simulink model "PPSFB_DC_DC_att_11"  (R2021a)
settings: Solver=ode23t  StartTime=0.0  StopTime=0.5  FixedStep=1.0000e-8  RelTol=1e-3
libraries: spsSeriesRLCBranchLib x31, spsVoltageMeasurementLib x9, spsMosfetLib x8, spsGroundLib x6, spsControlledVoltageSourceLib x3, spsCurrentMeasurementLib x2, spsLinearTransformerLib x2, pid_lib x2, spsParallelRLCBranchLib x2, spsDCVoltageSourceLib x1, spspowerguiLib x1
settings Model: Creator=prizm  LastModifiedBy=prizm

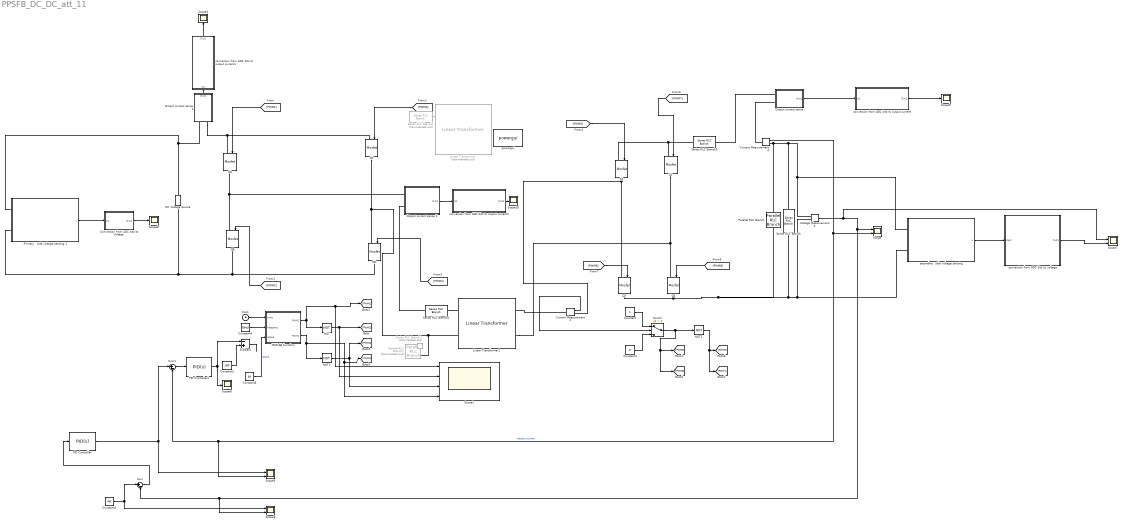
== system PPSFB_DC_DC_att_11 ==
  Clock : Clock
  Constant : Constant
  Constant1 : Constant  Value=0
  Constant2 : Constant  Value=180
  Constant3 : Constant  Value=48
  Constant4 : Constant  Value=65e3
  Constant5 : Constant  Value=90  SampleTime=1e-8
  "Conversion from ADC bits to Voltage " : Subsystem
  Current Measurement1 : spsCurrentMeasurementLib/Current Measurement  PhasorSimulation=off  OutputType=Complex  PSBequivalent=0
  Current Measurement4 : spsCurrentMeasurementLib/Current Measurement  PhasorSimulation=off  OutputType=Complex  PSBequivalent=0
  DC Voltage Source : spsDCVoltageSourceLib/DC Voltage Source  Amplitude=800  Measurements=None
  Linear Transformer : spsLinearTransformerLib/Linear Transformer  Commented=on  UNITS=SI  NominalPower=[5000 100000]  winding1=[750 0 0]  winding2=[107.25 0.003 300e-9]  ThreeWindings=off  winding3=[3.15e+05 0 0]  RmLm=[10e9 10.66e-3]  Measurements=None  DataType=on
  Linear Transformer1 : spsLinearTransformerLib/Linear Transformer  UNITS=SI  NominalPower=[5000 65000]  winding1=[800 0.245 10e-6]  winding2=[114 5e-3 1.143e-6]  ThreeWindings=off  winding3=[3.15e+05 0 0]  RmLm=[10e9 3.53e-3]  Measurements=None  DataType=on
  MATLAB Function : MATLAB Function  TreatAsAtomicUnit=on
  NOT : Logic  Operator=NOT  IconShape=distinctive  AllPortsSameDT=off  OutDataTypeStr=boolean
  NOT1 : Logic  Operator=NOT  IconShape=distinctive  AllPortsSameDT=off  OutDataTypeStr=boolean
  NOT2 : Logic  Operator=NOT  IconShape=distinctive  AllPortsSameDT=off  OutDataTypeStr=boolean
  "Output current sense " : Subsystem
  Output current sense 1 : Subsystem
  Output current sense 2 : Subsystem
  PID Controller : pid_lib/PID Controller  Controller=PID  Form=Parallel  TimeDomain=Continuous-time  UseExternalTs=off  SampleTime=-1  IntegratorMethod=Forward Euler  FilterMethod=Forward Euler  ControllerParametersSource=internal  P=0.003  I=100  D=0  UseFilter=on  N=100  TunerSelectOption=Frequency Response Based  InitialConditionSource=internal  InitialConditionForIntegrator=0  InitialConditionForFilter=0  DifferentiatorICPrevScaledInput=0  ExternalReset=none  TrackingMode=off  Kt=1  LimitOutput=on  SatLimitsSource=internal  UpperSaturationLimit=200  LowerSaturationLimit=0  LinearizeAsGain=on  AntiWindupMode=none  Kb=1  POutMin=[]  POutMax=[]  IOutMin=[]  IOutMax=[]  DOutMin=[]  DOutMax=[]  NOutMin=[]  NOutMax=[]  SumOutMin=[]  SumOutMax=[]  SaturationOutMin=[]  SaturationOutMax=[]  PParamMin=[]  PParamMax=[]  IParamMin=[]  IParamMax=[]  DParamMin=[]  DParamMax=[]  NParamMin=[]  NParamMax=[]  KbParamMin=[]  KbParamMax=[]  KtParamMin=[]  KtParamMax=[]  KbOutMin=[]  KbOutMax=[]  KtOutMin=[]  KtOutMax=[]  IntegratorOutMin=[]  IntegratorOutMax=[]  FilterOutMin=[]  FilterOutMax=[]  SumI1OutMin=[]  SumI1OutMax=[]  SumI2OutMin=[]  SumI2OutMax=[]  SumI3OutMin=[]  SumI3OutMax=[]  SumI4OutMin=[]  SumI4OutMax=[]  SumDOutMin=[]  SumDOutMax=[]  DifferentiatorOutMin=[]  DifferentiatorOutMax=[]  FilterDiffOutCoefMin=[]  FilterDiffOutCoefMax=[]  ReciprocalOutMin=[]  ReciprocalOutMax=[]  SumDenOutMin=[]  SumDenOutMax=[]  SumNumOutMin=[]  SumNumOutMax=[]  DivideOutMin=[]  DivideOutMax=[]  UdiffTsProdOutMin=[]  UdiffTsProdOutMax=[]  NTsProdOutMin=[]  NTsProdOutMax=[]  UintegralTsProdOutMin=[]  UintegralTsProdOutMax=[]  UngainTsProdOutMin=[]  UngainTsProdOutMax=[]  IntegratorContinuousStateAttributes=''  IntegratorStateMustResolveToSignalObject=off  IntegratorRTWStateStorageClass=Auto  FilterContinuousStateAttributes=''  FilterStateMustResolveToSignalObject=off  FilterRTWStateStorageClass=Auto  ParallelPVariant=InternalParameters  IdealPVariant=Disabled  IVariant=InternalParameters  DVariant=InternalParameters  IntegratorVariant=Continuous  SatVariant=Enabled  AWVariant=Passthrough  PCopyVariant=Disabled  TRVariant=Disabled  FdbkBlocksVariant=Forward  IdealPFdbkVariant=Disabled  SatFdbkVariant=Disabled  DerivativeFilterVariant=ContFilter  NVariant=InternalParameters  NCopyVariant=Disabled  FilterICVariant=InternalICsFilter  IntegratorICVariant=InternalICs  ExternalResetVariant=Disabled  TRSumVariant=Passthrough  SumFdbkVariant=Disabled  SumVariant=Sum_PID  TsampFilterVariant=InternalTs  TsampNgainVariant=Passthrough  TsampIntegralVariant=Passthrough  ExternalSaturationOutDataTypeStr=Inherit: Same as second input
  PID Controller1 : pid_lib/PID Controller  Controller=PID  Form=Parallel  TimeDomain=Continuous-time  UseExternalTs=off  SampleTime=-1  IntegratorMethod=Forward Euler  FilterMethod=Forward Euler  ControllerParametersSource=internal  P=0.074  I=942.478  D=0  UseFilter=on  N=100  TunerSelectOption=Transfer Function Based (PID Tuner App)  InitialConditionSource=internal  InitialConditionForIntegrator=0  InitialConditionForFilter=0  DifferentiatorICPrevScaledInput=0  ExternalReset=none  TrackingMode=off  Kt=1  LimitOutput=on  SatLimitsSource=internal  UpperSaturationLimit=180  LowerSaturationLimit=0  LinearizeAsGain=on  AntiWindupMode=none  Kb=1  POutMin=[]  POutMax=[]  IOutMin=[]  IOutMax=[]  DOutMin=[]  DOutMax=[]  NOutMin=[]  NOutMax=[]  SumOutMin=[]  SumOutMax=[]  SaturationOutMin=[]  SaturationOutMax=[]  PParamMin=[]  PParamMax=[]  IParamMin=[]  IParamMax=[]  DParamMin=[]  DParamMax=[]  NParamMin=[]  NParamMax=[]  KbParamMin=[]  KbParamMax=[]  KtParamMin=[]  KtParamMax=[]  KbOutMin=[]  KbOutMax=[]  KtOutMin=[]  KtOutMax=[]  IntegratorOutMin=[]  IntegratorOutMax=[]  FilterOutMin=[]  FilterOutMax=[]  SumI1OutMin=[]  SumI1OutMax=[]  SumI2OutMin=[]  SumI2OutMax=[]  SumI3OutMin=[]  SumI3OutMax=[]  SumI4OutMin=[]  SumI4OutMax=[]  SumDOutMin=[]  SumDOutMax=[]  DifferentiatorOutMin=[]  DifferentiatorOutMax=[]  FilterDiffOutCoefMin=[]  FilterDiffOutCoefMax=[]  ReciprocalOutMin=[]  ReciprocalOutMax=[]  SumDenOutMin=[]  SumDenOutMax=[]  SumNumOutMin=[]  SumNumOutMax=[]  DivideOutMin=[]  DivideOutMax=[]  UdiffTsProdOutMin=[]  UdiffTsProdOutMax=[]  NTsProdOutMin=[]  NTsProdOutMax=[]  UintegralTsProdOutMin=[]  UintegralTsProdOutMax=[]  UngainTsProdOutMin=[]  UngainTsProdOutMax=[]  IntegratorContinuousStateAttributes=''  IntegratorStateMustResolveToSignalObject=off  IntegratorRTWStateStorageClass=Auto  FilterContinuousStateAttributes=''  FilterStateMustResolveToSignalObject=off  FilterRTWStateStorageClass=Auto  ParallelPVariant=InternalParameters  IdealPVariant=Disabled  IVariant=InternalParameters  DVariant=InternalParameters  IntegratorVariant=Continuous  SatVariant=Enabled  AWVariant=Passthrough  PCopyVariant=Disabled  TRVariant=Disabled  FdbkBlocksVariant=Forward  IdealPFdbkVariant=Disabled  SatFdbkVariant=Disabled  DerivativeFilterVariant=ContFilter  NVariant=InternalParameters  NCopyVariant=Disabled  FilterICVariant=InternalICsFilter  IntegratorICVariant=InternalICs  ExternalResetVariant=Disabled  TRSumVariant=Passthrough  SumFdbkVariant=Disabled  SumVariant=Sum_PID  TsampFilterVariant=InternalTs  TsampNgainVariant=Passthrough  TsampIntegralVariant=Passthrough  ExternalSaturationOutDataTypeStr=Inherit: Same as second input
  Parallel RLC Branch : spsParallelRLCBranchLib/Parallel RLC Branch  LConnTagsString=a  RConnTagsString=__new0  BranchType=R  Resistance=0.461  Inductance=1e-3  SetiL0=off  InitialCurrent=0  Capacitance=1e-6  Setx0=off  InitialVoltage=0  Measurements=None
  Parallel RLC Branch1 : spsParallelRLCBranchLib/Parallel RLC Branch  Commented=on  LConnTagsString=a  RConnTagsString=__new0  BranchType=L  Resistance=100  Inductance=1.88e-6  SetiL0=off  InitialCurrent=0  Capacitance=1e-6  Setx0=off  InitialVoltage=0  Measurements=None
  Primary   side voltage sensing 1 : Subsystem
  Q{1..4} (4 alike) : spsMosfetLib/Mosfet  Ron=0.1  Lon=0  Rd=0.01  Vfd=2  IC=0  Rs=1e5  Cs=inf  Measurements=off
  QA : spsMosfetLib/Mosfet  Ron=0.1  Lon=0  Rd=0.01  Vfd=2  IC=0  Rs=1e5  Cs=inf  Measurements=off
  QB : spsMosfetLib/Mosfet  Ron=0.1  Lon=0  Rd=0.01  Vfd=2  IC=0  Rs=1e5  Cs=inf  Measurements=off
  QC : spsMosfetLib/Mosfet  Ron=0.1  Lon=0  Rd=0.01  Vfd=2  IC=0  Rs=1e5  Cs=inf  Measurements=off
  QD : spsMosfetLib/Mosfet  Ron=0.1  Lon=0  Rd=0.01  Vfd=2  IC=0  Rs=1e5  Cs=inf  Measurements=off
  Scope{,3,5,7} (4 alike) : Scope  NumInputPorts=2
  Scope1 : Scope  NumInputPorts=4
  Scope{4,6,8..10} (5 alike) : Scope
  Series RLC Branch : spsSeriesRLCBranchLib/Series RLC Branch  LConnTagsString=__new0  RConnTagsString=__new0  BranchType=C  Resistance=1  Inductance=1e-3  SetiL0=off  InitialCurrent=0  Capacitance=1e-3  Setx0=off  InitialVoltage=0  Measurements=None
  Series RLC Branch1 : spsSeriesRLCBranchLib/Series RLC Branch  Commented=on  LConnTagsString=__new0  RConnTagsString=__new0  BranchType=RL  Resistance=0.126  Inductance=10e-6  SetiL0=off  InitialCurrent=0  Capacitance=1e-6  Setx0=off  InitialVoltage=0  Measurements=None
  Series RLC Branch2 : spsSeriesRLCBranchLib/Series RLC Branch  Commented=on  LConnTagsString=__new0  RConnTagsString=__new0  BranchType=C  Resistance=1  Inductance=1e-3  SetiL0=off  InitialCurrent=0  Capacitance=200e-12  Setx0=off  InitialVoltage=0  Measurements=None
  Series RLC Branch3 : spsSeriesRLCBranchLib/Series RLC Branch  LConnTagsString=__new0  RConnTagsString=__new0  BranchType=L  Resistance=0.005  Inductance=10e-6  SetiL0=off  InitialCurrent=0  Capacitance=1e-6  Setx0=off  InitialVoltage=0  Measurements=None
  Series RLC Branch4 : spsSeriesRLCBranchLib/Series RLC Branch  LConnTagsString=__new0  RConnTagsString=__new0  BranchType=L  Resistance=1  Inductance=20e-6  SetiL0=off  InitialCurrent=0  Capacitance=1e-6  Setx0=off  InitialVoltage=0  Measurements=None
  Subtract : Sum  Inputs=-+
  Sum : Sum  Inputs=|+-
  Sum1 : Sum  Inputs=|+-
  Switch : Switch  Criteria=u2 > Threshold
  Voltage Measurement2 : spsVoltageMeasurementLib/Voltage Measurement  PhasorSimulation=off  OutputType=Complex  PSBequivalent=0
  conversion from ADC bits to output current : Subsystem
  conversion from ADC bits to output current1 : Subsystem
  conversion from ADC bits to output current2 : Subsystem
  "conversion from ADC bits to voltage " : Subsystem
  powergui : spspowerguiLib/powergui  Priority=1  SimulationMode=Discrete  SampleTime=1e-8  frequency=60  Iterations=50  frequencyindice=0  Pbase=100e6  ErrMax=1e-4  UnitsV=kV  UnitsW=MW  buscounter=0  FunctionMessages=off  echomessages=off  EnableUseOfTLC=off  CurrentSourceSwitches=off  DisableSnubberDevices=off  DisableRonSwitches=off  DisableVfSwitches=off  DisplayEquations=off  AutomaticDiscreteSolvers=off  SolverType=Tustin/Backward Euler (TBE)  Interpol=off  ExternalGateDelay=off  methode=off  Ts=100  x0status=blocks  SPID=on  SwTol=0  HookPort=off  NonlinearTolerance=1e-4  nMaxIteration=100  ContinueOnMaxIteration=off  RestoreLinks=warning  ResistiveCurrentMeasurement=off  Frange=[0:2:500]  Ylog=off  Xlog=on  ShowGrid=off  save=off  variable=ZData  structure=0  ZoomFFT=off  StartTime=0.0  cycles=1  DisplayStyle=1  fundamental=60  FreqAxis=off  MaxFrequency=1000  frequencyindicesteady=1  RmsSteady=1  display=off
  "secondary  side voltage sensing " : Subsystem
  wires:
  Current Measurement1/1 -> Switch/2
  Constant/1 -> Switch/1
  Constant1/1 -> Switch/3
  Voltage Measurement2/1 -> Scope7/1, Scope3/2, Sum/2, Scope/1
  Constant3/1 -> Sum/1, Scope3/1
  Constant4/1 -> MATLAB Function/2(frequency)
  Clock/1 -> MATLAB Function/1(time)
  MATLAB Function/1(PWM2) -> NOT/1, Scope1/1, [PWM1]
  MATLAB Function/2(PWM1) -> [PWM4], Scope1/4, NOT1/1
  [PWM1] -> QA/1
  [PWM2] -> QB/1
  [PWM3] -> QC/1
  [PWM4] -> QD/1
  NOT/1 -> Scope1/2, [PWM2]
  NOT1/1 -> [PWM3], Scope1/3
  [PWM5] -> Q1/1
  [PWM8] -> Q4/1
  Switch/1 -> [PWM5], [PWM8], NOT2/1
  NOT2/1 -> [PWM6], [PWM7]
  [PWM7] -> Q2/1
  [PWM6] -> Q3/1
  Constant2/1 -> Subtract/2
  Subtract/1 -> ?
  Sum1/1 -> PID Controller1/1
  Current Measurement4/1 -> Scope5/2, Sum1/2, Scope/2  "inductor current"
  PID Controller1/1 -> Scope6/1, Subtract/1
  PID Controller/1 -> Sum1/1, Scope5/1
  Sum/1 -> PID Controller/1
  "secondary  side voltage sensing "/1(v) -> "conversion from ADC bits to voltage "/1(Input)
  Primary   side voltage sensing 1/1(v) -> "Conversion from ADC bits to Voltage "/1(In1)
  "conversion from ADC bits to voltage "/1(Out1) -> Scope7/2
  "Conversion from ADC bits to Voltage "/1(Out1) -> Scope8/1
  "Output current sense "/1(Out1) -> conversion from ADC bits to output current/1(In1)
  conversion from ADC bits to output current/1(Out1) -> Scope9/1
  Output current sense 2/1(Out1) -> conversion from ADC bits to output current2/1(In1)
  Output current sense 1/1(Out1) -> conversion from ADC bits to output current1/1(In1)
  conversion from ADC bits to output current1/1(Out1) -> Scope4/1
  conversion from ADC bits to output current2/1(Out1) -> Scope10/1
  Constant5/1 -> MATLAB Function/3(phase)  "phase"
  connections:
  DC Voltage Source/RConn1 -- Primary   side voltage sensing 1/LConn1 -- Output current sense 1/LConn1
  QC/RConn1 -- Linear Transformer1/LConn2 -- Series RLC Branch2/RConn1 -- QD/LConn1
  Current Measurement4/RConn1 -- Voltage Measurement2/LConn1 -- "secondary  side voltage sensing "/LConn1 -- Series RLC Branch/LConn1 -- Parallel RLC Branch/LConn1
  Q3/RConn1 -- Voltage Measurement2/LConn2 -- "secondary  side voltage sensing "/LConn2 -- Series RLC Branch/RConn1 -- Parallel RLC Branch/RConn1 -- Q4/RConn1
  Q1/RConn1 -- Current Measurement1/RConn1 -- Q3/LConn1
  Q1/LConn1 -- Q2/LConn1 -- Series RLC Branch3/LConn1
  Current Measurement1/LConn1 -- Linear Transformer1/RConn1
  Output current sense 2/LConn2 -- Series RLC Branch4/LConn1
  "Output current sense "/LConn1 -- Series RLC Branch3/RConn1
  Current Measurement4/LConn1 -- "Output current sense "/LConn2
  Series RLC Branch1/RConn1 -- Linear Transformer/LConn1
  Linear Transformer1/RConn2 -- Q2/RConn1 -- Q4/LConn1
  Series RLC Branch4/RConn1 -- Linear Transformer1/LConn1
  QB/RConn1 -- DC Voltage Source/LConn1 -- Primary   side voltage sensing 1/LConn2 -- QD/RConn1
  Output current sense 2/LConn1 -- QB/LConn1 -- QA/RConn1
  QC/LConn1 -- Output current sense 1/LConn2 -- QA/LConn1

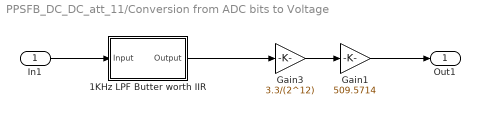
== system PPSFB_DC_DC_att_11/Conversion from ADC bits to Voltage  ==
  In1 : Inport
  "1KHz LPF Butter worth IIR " : Subsystem  Tag=FilterWizardSubSystem
      settings: ErrorFcn=dspFilterRealizedInBasicElemsAlgLoopErrFcnCallback
  Gain1 : Gain  Gain=509.5714
  Gain3 : Gain  Gain=3.3/(2^12)
  Out1 : Outport
  wires:
  Gain1/1 -> Out1/1
  Gain3/1 -> Gain1/1
  In1/1 -> "1KHz LPF Butter worth IIR "/1(Input)
  "1KHz LPF Butter worth IIR "/1(Output) -> Gain3/1

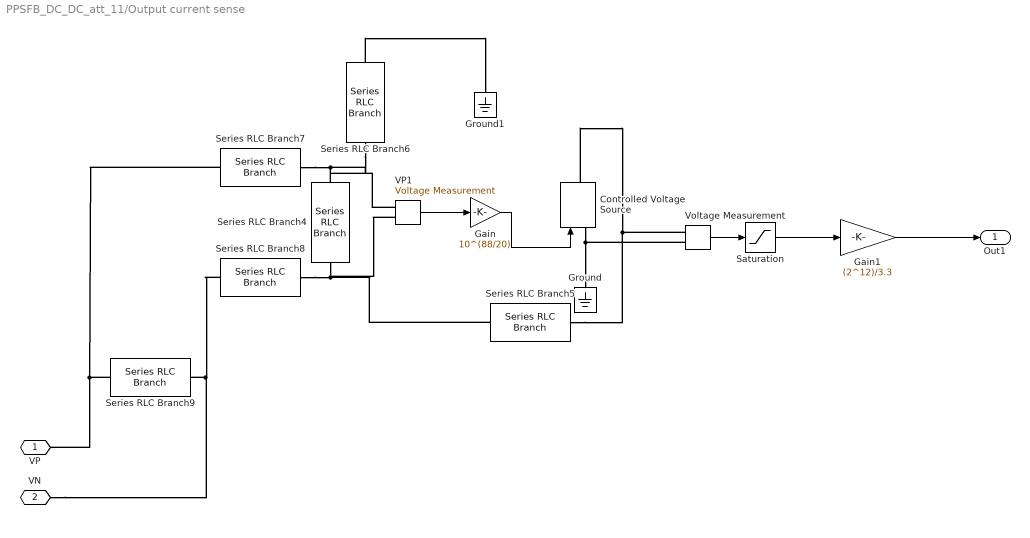
== system PPSFB_DC_DC_att_11/Output current sense  ==
  Controlled Voltage Source : spsControlledVoltageSourceLib/Controlled Voltage Source  Initialize=on  Source_Type=AC  Amplitude=0  Phase=0  Frequency=0  Measurements=None
  Gain : Gain  Gain=10^(88/20)
  Gain1 : Gain  Gain=(2^12)/3.3
  Ground : spsGroundLib/Ground  LConnTagsString=a
  Ground1 : spsGroundLib/Ground  LConnTagsString=a
  Saturation : Saturate  UpperLimit=3.3  LowerLimit=0
  Series RLC Branch4 : spsSeriesRLCBranchLib/Series RLC Branch  LConnTagsString=__new0  RConnTagsString=__new0  BranchType=R  Resistance=10e6  Inductance=1e-3  SetiL0=off  InitialCurrent=0  Capacitance=1e-6  Setx0=off  InitialVoltage=0  Measurements=None
  Series RLC Branch5 : spsSeriesRLCBranchLib/Series RLC Branch  LConnTagsString=__new0  RConnTagsString=__new0  BranchType=R  Resistance=390e3  Inductance=1e-3  SetiL0=off  InitialCurrent=0  Capacitance=1e-6  Setx0=off  InitialVoltage=0  Measurements=None
  Series RLC Branch6 : spsSeriesRLCBranchLib/Series RLC Branch  LConnTagsString=__new0  RConnTagsString=__new0  BranchType=R  Resistance=390e3  Inductance=1e-3  SetiL0=off  InitialCurrent=0  Capacitance=1e-6  Setx0=off  InitialVoltage=0  Measurements=None
  Series RLC Branch7 : spsSeriesRLCBranchLib/Series RLC Branch  LConnTagsString=__new0  RConnTagsString=__new0  BranchType=R  Resistance=8.2e3  Inductance=1e-3  SetiL0=off  InitialCurrent=0  Capacitance=1e-6  Setx0=off  InitialVoltage=0  Measurements=None
  Series RLC Branch8 : spsSeriesRLCBranchLib/Series RLC Branch  LConnTagsString=__new0  RConnTagsString=__new0  BranchType=R  Resistance=8.2e3  Inductance=1e-3  SetiL0=off  InitialCurrent=0  Capacitance=1e-6  Setx0=off  InitialVoltage=0  Measurements=None
  Series RLC Branch9 : spsSeriesRLCBranchLib/Series RLC Branch  LConnTagsString=__new0  RConnTagsString=__new0  BranchType=R  Resistance=0.0001  Inductance=10e-6  SetiL0=off  InitialCurrent=0  Capacitance=1e-6  Setx0=off  InitialVoltage=0  Measurements=None
  VP1 : spsVoltageMeasurementLib/Voltage Measurement  PhasorSimulation=off  OutputType=Complex  PSBequivalent=0
  Voltage Measurement : spsVoltageMeasurementLib/Voltage Measurement  PhasorSimulation=off  OutputType=Complex  PSBequivalent=0
  VP : PMIOPort  Side=Left
  VN : PMIOPort  Port=2  Side=Left
  Out1 : Outport
  wires:
  Voltage Measurement/1 -> Saturation/1
  Gain/1 -> Controlled Voltage Source/1
  VP1/1 -> Gain/1
  Saturation/1 -> Gain1/1
  Gain1/1 -> Out1/1
  connections:
  Series RLC Branch4/LConn1 -- Series RLC Branch6/LConn1 -- VP1/LConn1 -- Series RLC Branch7/LConn1
  Series RLC Branch6/RConn1 -- Ground1/LConn1
  Controlled Voltage Source/RConn1 -- Voltage Measurement/LConn1 -- Series RLC Branch5/LConn1
  Controlled Voltage Source/LConn1 -- Ground/LConn1 -- Voltage Measurement/LConn2
  Series RLC Branch4/RConn1 -- Series RLC Branch5/RConn1 -- VP1/LConn2 -- Series RLC Branch8/LConn1
  Series RLC Branch9/LConn1 -- VP/RConn1 -- Series RLC Branch7/RConn1
  Series RLC Branch9/RConn1 -- VN/RConn1 -- Series RLC Branch8/RConn1

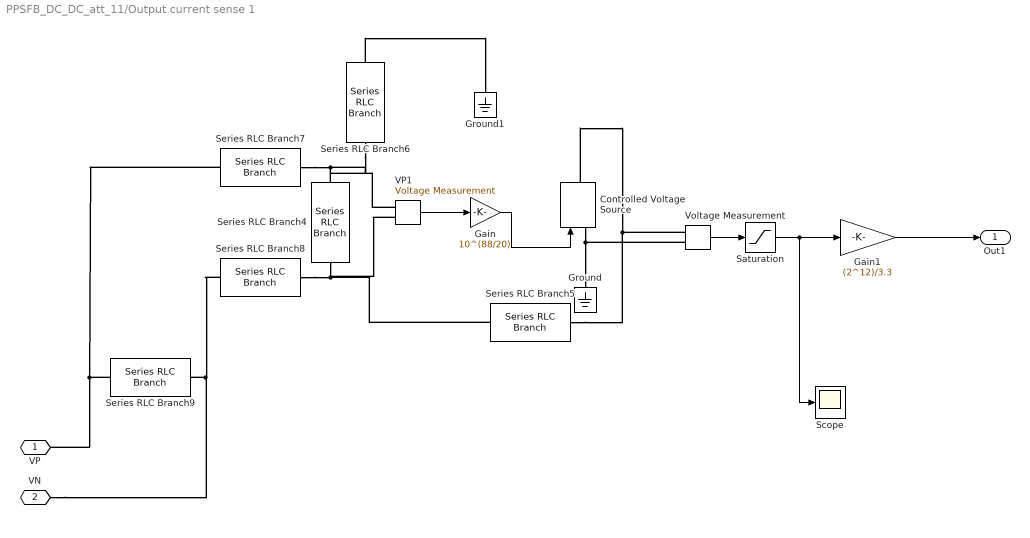
== system PPSFB_DC_DC_att_11/Output current sense 1 ==
  Controlled Voltage Source : spsControlledVoltageSourceLib/Controlled Voltage Source  Initialize=on  Source_Type=AC  Amplitude=0  Phase=0  Frequency=0  Measurements=None
  Gain : Gain  Gain=10^(88/20)
  Gain1 : Gain  Gain=(2^12)/3.3
  Ground : spsGroundLib/Ground  LConnTagsString=a
  Ground1 : spsGroundLib/Ground  LConnTagsString=a
  Saturation : Saturate  UpperLimit=3.3  LowerLimit=0
  Scope : Scope
  Series RLC Branch4 : spsSeriesRLCBranchLib/Series RLC Branch  LConnTagsString=__new0  RConnTagsString=__new0  BranchType=R  Resistance=10e6  Inductance=1e-3  SetiL0=off  InitialCurrent=0  Capacitance=1e-6  Setx0=off  InitialVoltage=0  Measurements=None
  Series RLC Branch5 : spsSeriesRLCBranchLib/Series RLC Branch  LConnTagsString=__new0  RConnTagsString=__new0  BranchType=R  Resistance=100e3  Inductance=1e-3  SetiL0=off  InitialCurrent=0  Capacitance=1e-6  Setx0=off  InitialVoltage=0  Measurements=None
  Series RLC Branch6 : spsSeriesRLCBranchLib/Series RLC Branch  LConnTagsString=__new0  RConnTagsString=__new0  BranchType=R  Resistance=100e3  Inductance=1e-3  SetiL0=off  InitialCurrent=0  Capacitance=1e-6  Setx0=off  InitialVoltage=0  Measurements=None
  Series RLC Branch7 : spsSeriesRLCBranchLib/Series RLC Branch  LConnTagsString=__new0  RConnTagsString=__new0  BranchType=R  Resistance=1.5e3  Inductance=1e-3  SetiL0=off  InitialCurrent=0  Capacitance=1e-6  Setx0=off  InitialVoltage=0  Measurements=None
  Series RLC Branch8 : spsSeriesRLCBranchLib/Series RLC Branch  LConnTagsString=__new0  RConnTagsString=__new0  BranchType=R  Resistance=1.5e3  Inductance=1e-3  SetiL0=off  InitialCurrent=0  Capacitance=1e-6  Setx0=off  InitialVoltage=0  Measurements=None
  Series RLC Branch9 : spsSeriesRLCBranchLib/Series RLC Branch  LConnTagsString=__new0  RConnTagsString=__new0  BranchType=R  Resistance=0.0001  Inductance=10e-6  SetiL0=off  InitialCurrent=0  Capacitance=1e-6  Setx0=off  InitialVoltage=0  Measurements=None
  VP1 : spsVoltageMeasurementLib/Voltage Measurement  PhasorSimulation=off  OutputType=Complex  PSBequivalent=0
  Voltage Measurement : spsVoltageMeasurementLib/Voltage Measurement  PhasorSimulation=off  OutputType=Complex  PSBequivalent=0
  VP : PMIOPort  Side=Left
  VN : PMIOPort  Port=2  Side=Left
  Out1 : Outport
  wires:
  Voltage Measurement/1 -> Saturation/1
  Gain/1 -> Controlled Voltage Source/1
  VP1/1 -> Gain/1
  Saturation/1 -> Scope/1, Gain1/1
  Gain1/1 -> Out1/1
  connections:
  Series RLC Branch4/LConn1 -- Series RLC Branch6/LConn1 -- VP1/LConn1 -- Series RLC Branch7/LConn1
  Series RLC Branch6/RConn1 -- Ground1/LConn1
  Controlled Voltage Source/RConn1 -- Voltage Measurement/LConn1 -- Series RLC Branch5/LConn1
  Controlled Voltage Source/LConn1 -- Ground/LConn1 -- Voltage Measurement/LConn2
  Series RLC Branch4/RConn1 -- Series RLC Branch5/RConn1 -- VP1/LConn2 -- Series RLC Branch8/LConn1
  Series RLC Branch9/LConn1 -- VP/RConn1 -- Series RLC Branch7/RConn1
  Series RLC Branch9/RConn1 -- VN/RConn1 -- Series RLC Branch8/RConn1

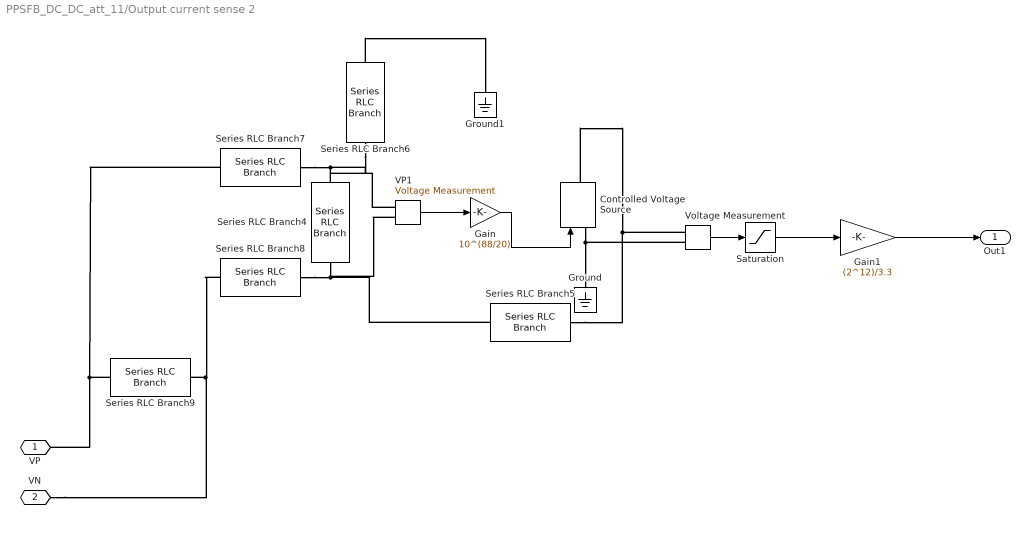
== system PPSFB_DC_DC_att_11/Output current sense 2 ==
  Controlled Voltage Source : spsControlledVoltageSourceLib/Controlled Voltage Source  Initialize=on  Source_Type=AC  Amplitude=0  Phase=0  Frequency=0  Measurements=None
  Gain : Gain  Gain=10^(88/20)
  Gain1 : Gain  Gain=(2^12)/3.3
  Ground : spsGroundLib/Ground  LConnTagsString=a
  Ground1 : spsGroundLib/Ground  LConnTagsString=a
  Saturation : Saturate  UpperLimit=3.3  LowerLimit=0
  Series RLC Branch4 : spsSeriesRLCBranchLib/Series RLC Branch  LConnTagsString=__new0  RConnTagsString=__new0  BranchType=R  Resistance=10e6  Inductance=1e-3  SetiL0=off  InitialCurrent=0  Capacitance=1e-6  Setx0=off  InitialVoltage=0  Measurements=None
  Series RLC Branch5 : spsSeriesRLCBranchLib/Series RLC Branch  LConnTagsString=__new0  RConnTagsString=__new0  BranchType=R  Resistance=100e3  Inductance=1e-3  SetiL0=off  InitialCurrent=0  Capacitance=1e-6  Setx0=off  InitialVoltage=0  Measurements=None
  Series RLC Branch6 : spsSeriesRLCBranchLib/Series RLC Branch  LConnTagsString=__new0  RConnTagsString=__new0  BranchType=R  Resistance=100e3  Inductance=1e-3  SetiL0=off  InitialCurrent=0  Capacitance=1e-6  Setx0=off  InitialVoltage=0  Measurements=None
  Series RLC Branch7 : spsSeriesRLCBranchLib/Series RLC Branch  LConnTagsString=__new0  RConnTagsString=__new0  BranchType=R  Resistance=1.5e3  Inductance=1e-3  SetiL0=off  InitialCurrent=0  Capacitance=1e-6  Setx0=off  InitialVoltage=0  Measurements=None
  Series RLC Branch8 : spsSeriesRLCBranchLib/Series RLC Branch  LConnTagsString=__new0  RConnTagsString=__new0  BranchType=R  Resistance=1.5e3  Inductance=1e-3  SetiL0=off  InitialCurrent=0  Capacitance=1e-6  Setx0=off  InitialVoltage=0  Measurements=None
  Series RLC Branch9 : spsSeriesRLCBranchLib/Series RLC Branch  LConnTagsString=__new0  RConnTagsString=__new0  BranchType=R  Resistance=0.0001  Inductance=10e-6  SetiL0=off  InitialCurrent=0  Capacitance=1e-6  Setx0=off  InitialVoltage=0  Measurements=None
  VP1 : spsVoltageMeasurementLib/Voltage Measurement  PhasorSimulation=off  OutputType=Complex  PSBequivalent=0
  Voltage Measurement : spsVoltageMeasurementLib/Voltage Measurement  PhasorSimulation=off  OutputType=Complex  PSBequivalent=0
  VP : PMIOPort  Side=Left
  VN : PMIOPort  Port=2  Side=Left
  Out1 : Outport
  wires:
  Voltage Measurement/1 -> Saturation/1
  Gain/1 -> Controlled Voltage Source/1
  VP1/1 -> Gain/1
  Saturation/1 -> Gain1/1
  Gain1/1 -> Out1/1
  connections:
  Series RLC Branch4/LConn1 -- Series RLC Branch6/LConn1 -- VP1/LConn1 -- Series RLC Branch7/LConn1
  Series RLC Branch6/RConn1 -- Ground1/LConn1
  Controlled Voltage Source/RConn1 -- Voltage Measurement/LConn1 -- Series RLC Branch5/LConn1
  Controlled Voltage Source/LConn1 -- Ground/LConn1 -- Voltage Measurement/LConn2
  Series RLC Branch4/RConn1 -- Series RLC Branch5/RConn1 -- VP1/LConn2 -- Series RLC Branch8/LConn1
  Series RLC Branch9/LConn1 -- VP/RConn1 -- Series RLC Branch7/RConn1
  Series RLC Branch9/RConn1 -- VN/RConn1 -- Series RLC Branch8/RConn1

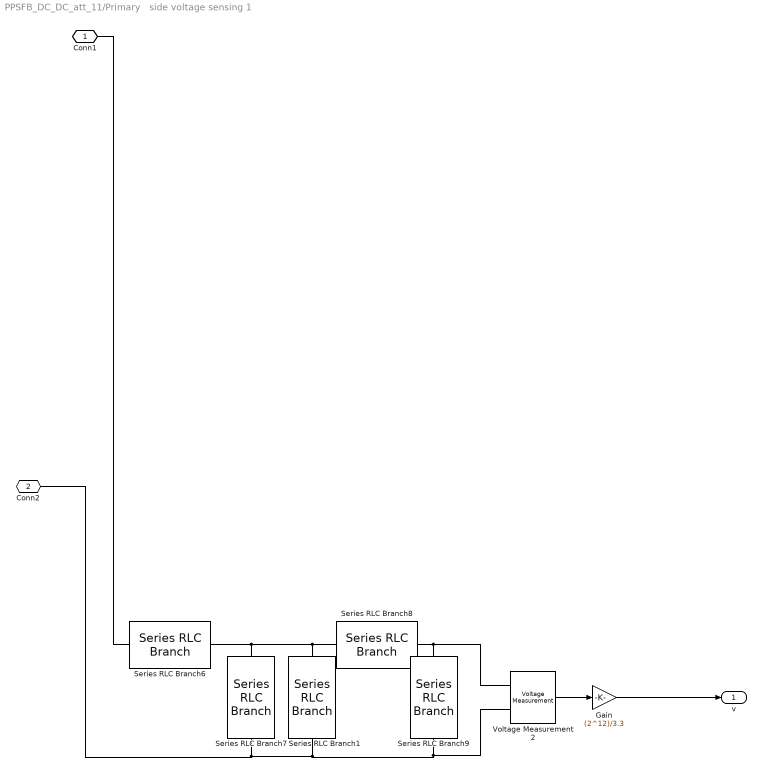
== system PPSFB_DC_DC_att_11/Primary   side voltage sensing 1 ==
  Gain : Gain  Gain=(2^12)/3.3
  Series RLC Branch1 : spsSeriesRLCBranchLib/Series RLC Branch  LConnTagsString=__new0  RConnTagsString=__new0  BranchType=C  Resistance=54.0  Inductance=0.2533e-3  SetiL0=off  InitialCurrent=0  Capacitance=0.2e-12  Setx0=off  InitialVoltage=0  Measurements=None
  Series RLC Branch6 : spsSeriesRLCBranchLib/Series RLC Branch  LConnTagsString=__new0  RConnTagsString=__new0  BranchType=R  Resistance=10.68e6  Inductance=0.2533e-3  SetiL0=off  InitialCurrent=0  Capacitance=1e-6  Setx0=off  InitialVoltage=0  Measurements=None
  Series RLC Branch7 : spsSeriesRLCBranchLib/Series RLC Branch  LConnTagsString=__new0  RConnTagsString=__new0  BranchType=R  Resistance=21e3  Inductance=0.2533e-3  SetiL0=off  InitialCurrent=0  Capacitance=1e-6  Setx0=off  InitialVoltage=0  Measurements=None
  Series RLC Branch8 : spsSeriesRLCBranchLib/Series RLC Branch  LConnTagsString=__new0  RConnTagsString=__new0  BranchType=R  Resistance=10e3  Inductance=0.2533e-3  SetiL0=off  InitialCurrent=0  Capacitance=1e-6  Setx0=off  InitialVoltage=0  Measurements=None
  Series RLC Branch9 : spsSeriesRLCBranchLib/Series RLC Branch  LConnTagsString=__new0  RConnTagsString=__new0  BranchType=C  Resistance=54.0  Inductance=0.2533e-3  SetiL0=off  InitialCurrent=0  Capacitance=100e-12  Setx0=off  InitialVoltage=0  Measurements=None
  Voltage Measurement2 : spsVoltageMeasurementLib/Voltage Measurement  PhasorSimulation=off  OutputType=Complex  PSBequivalent=0
  Conn1 : PMIOPort  Side=Left
  Conn2 : PMIOPort  Port=2  Side=Left
  v : Outport
  wires:
  Voltage Measurement2/1 -> Gain/1
  Gain/1 -> v/1
  connections:
  Conn2/RConn1 -- Voltage Measurement2/LConn2 -- Series RLC Branch9/RConn1 -- Series RLC Branch1/RConn1 -- Series RLC Branch7/RConn1
  Series RLC Branch8/LConn1 -- Voltage Measurement2/LConn1 -- Series RLC Branch9/LConn1
  Conn1/RConn1 -- Series RLC Branch6/LConn1
  Series RLC Branch6/RConn1 -- Series RLC Branch8/RConn1 -- Series RLC Branch1/LConn1 -- Series RLC Branch7/LConn1

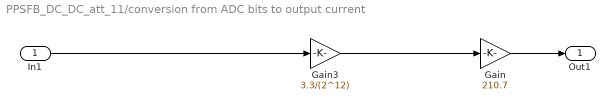
== system PPSFB_DC_DC_att_11/conversion from ADC bits to output current ==
  In1 : Inport
  Gain : Gain  Gain=210.7
  Gain3 : Gain  Gain=3.3/(2^12)
  Out1 : Outport
  wires:
  In1/1 -> Gain3/1
  Gain3/1 -> Gain/1
  Gain/1 -> Out1/1

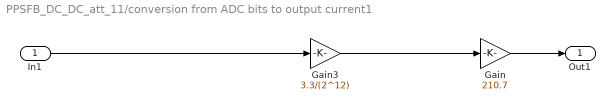
== system PPSFB_DC_DC_att_11/conversion from ADC bits to output current1 ==
  In1 : Inport
  Gain : Gain  Gain=210.7
  Gain3 : Gain  Gain=3.3/(2^12)
  Out1 : Outport
  wires:
  In1/1 -> Gain3/1
  Gain3/1 -> Gain/1
  Gain/1 -> Out1/1

== system PPSFB_DC_DC_att_11/conversion from ADC bits to output current2 ==
  In1 : Inport
  Gain : Gain  Gain=210.7
  Gain3 : Gain  Gain=3.3/(2^12)
  Out1 : Outport
  wires:
  In1/1 -> Gain3/1
  Gain3/1 -> Gain/1
  Gain/1 -> Out1/1

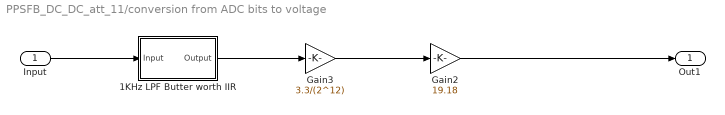
== system PPSFB_DC_DC_att_11/conversion from ADC bits to voltage  ==
  Input : Inport
  "1KHz LPF Butter worth IIR " : Subsystem  Tag=FilterWizardSubSystem
      settings: ErrorFcn=dspFilterRealizedInBasicElemsAlgLoopErrFcnCallback
  Gain2 : Gain  Gain=19.18
  Gain3 : Gain  Gain=3.3/(2^12)
  Out1 : Outport
  wires:
  Gain3/1 -> Gain2/1
  Gain2/1 -> Out1/1
  Input/1 -> "1KHz LPF Butter worth IIR "/1(Input)
  "1KHz LPF Butter worth IIR "/1(Output) -> Gain3/1

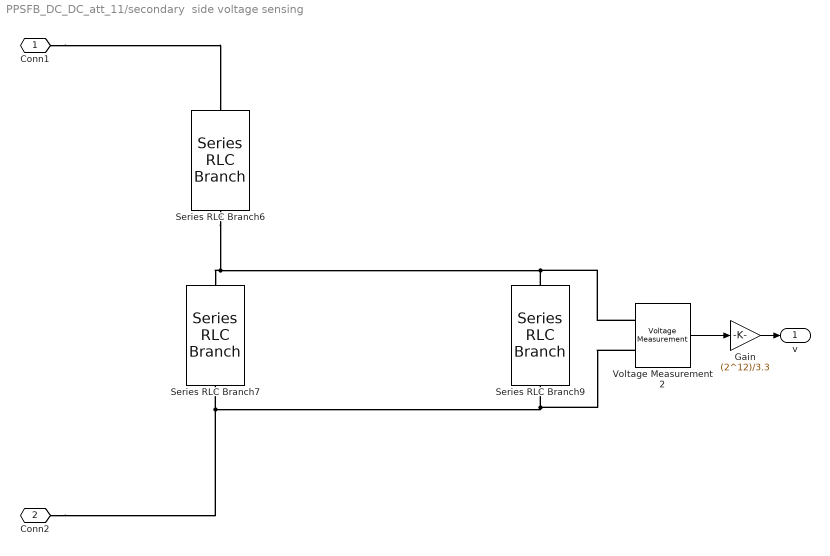
== system PPSFB_DC_DC_att_11/secondary  side voltage sensing  ==
  Gain : Gain  Gain=(2^12)/3.3
  Series RLC Branch6 : spsSeriesRLCBranchLib/Series RLC Branch  LConnTagsString=__new0  RConnTagsString=__new0  BranchType=R  Resistance=200e3  Inductance=0.2533e-3  SetiL0=off  InitialCurrent=0  Capacitance=1e-6  Setx0=off  InitialVoltage=0  Measurements=None
  Series RLC Branch7 : spsSeriesRLCBranchLib/Series RLC Branch  LConnTagsString=__new0  RConnTagsString=__new0  BranchType=R  Resistance=11e3  Inductance=0.2533e-3  SetiL0=off  InitialCurrent=0  Capacitance=1e-6  Setx0=off  InitialVoltage=0  Measurements=None
  Series RLC Branch9 : spsSeriesRLCBranchLib/Series RLC Branch  LConnTagsString=__new0  RConnTagsString=__new0  BranchType=C  Resistance=54.0  Inductance=0.2533e-3  SetiL0=off  InitialCurrent=0  Capacitance=100e-12  Setx0=off  InitialVoltage=0  Measurements=None
  Voltage Measurement2 : spsVoltageMeasurementLib/Voltage Measurement  PhasorSimulation=off  OutputType=Complex  PSBequivalent=0
  Conn1 : PMIOPort  Side=Left
  Conn2 : PMIOPort  Port=2  Side=Left
  v : Outport
  wires:
  Voltage Measurement2/1 -> Gain/1
  Gain/1 -> v/1
  connections:
  Series RLC Branch7/RConn1 -- Conn2/RConn1 -- Voltage Measurement2/LConn2 -- Series RLC Branch9/RConn1
  Series RLC Branch6/RConn1 -- Voltage Measurement2/LConn1 -- Series RLC Branch9/LConn1 -- Series RLC Branch7/LConn1
  Conn1/RConn1 -- Series RLC Branch6/LConn1

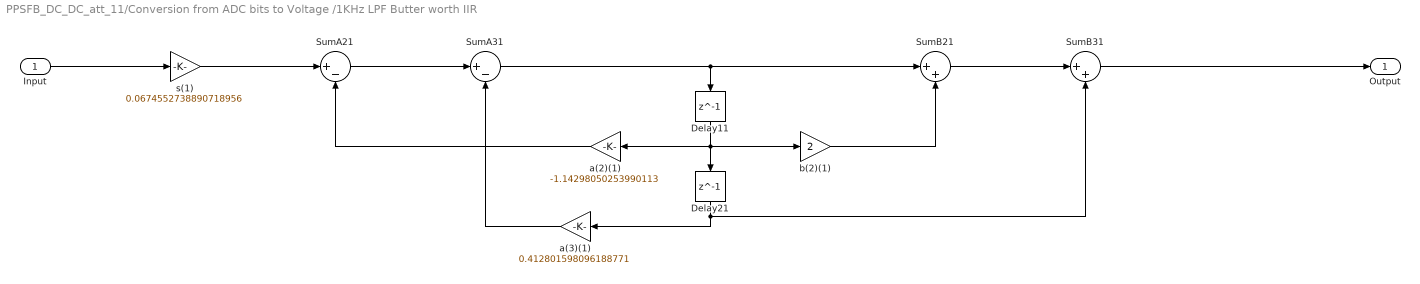
== system PPSFB_DC_DC_att_11/Conversion from ADC bits to Voltage /1KHz LPF Butter worth IIR  ==
  Input : Inport
  Delay11 : Delay  DelayLength=1  InitialCondition=0
  Delay21 : Delay  DelayLength=1  InitialCondition=0
  SumA21 : Sum  Inputs=|+-  RndMeth=Nearest  SaturateOnIntegerOverflow=on  OutDataTypeStr=Inherit: Same as first input
  SumA31 : Sum  Inputs=|+-  RndMeth=Nearest  SaturateOnIntegerOverflow=on  OutDataTypeStr=Inherit: Same as first input
  SumB21 : Sum  Inputs=|++  RndMeth=Nearest  SaturateOnIntegerOverflow=on  OutDataTypeStr=Inherit: Same as first input
  SumB31 : Sum  Inputs=|++  RndMeth=Nearest  SaturateOnIntegerOverflow=on  OutDataTypeStr=Inherit: Same as first input
  a(2)(1) : Gain  Gain=-1.14298050253990113  ParamDataTypeStr=double  RndMeth=Nearest  SaturateOnIntegerOverflow=on  OutDataTypeStr=Inherit: Same as input
  a(3)(1) : Gain  Gain=0.412801598096188771  ParamDataTypeStr=double  RndMeth=Nearest  SaturateOnIntegerOverflow=on  OutDataTypeStr=Inherit: Same as input
  b(2)(1) : Gain  Gain=2  ParamDataTypeStr=double  RndMeth=Nearest  SaturateOnIntegerOverflow=on  OutDataTypeStr=Inherit: Same as input
  s(1) : Gain  Gain=0.0674552738890718956  ParamDataTypeStr=double  RndMeth=Nearest  SaturateOnIntegerOverflow=on  OutDataTypeStr=Inherit: Same as input
  Output : Outport
  wires:
  Input/1 -> s(1)/1
  s(1)/1 -> SumA21/1
  SumA21/1 -> SumA31/1
  SumA31/1 -> SumB21/1, Delay11/1
  SumB21/1 -> SumB31/1
  SumB31/1 -> Output/1
  a(2)(1)/1 -> SumA21/2
  Delay11/1 -> a(2)(1)/1, b(2)(1)/1, Delay21/1
  b(2)(1)/1 -> SumB21/2
  a(3)(1)/1 -> SumA31/2
  Delay21/1 -> a(3)(1)/1, SumB31/2

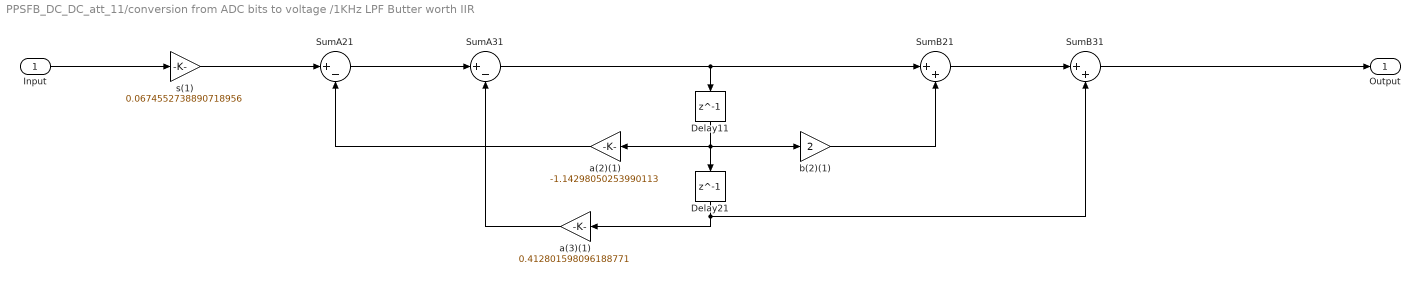
== system PPSFB_DC_DC_att_11/conversion from ADC bits to voltage /1KHz LPF Butter worth IIR  ==
  Input : Inport
  Delay11 : Delay  DelayLength=1  InitialCondition=0
  Delay21 : Delay  DelayLength=1  InitialCondition=0
  SumA21 : Sum  Inputs=|+-  RndMeth=Nearest  SaturateOnIntegerOverflow=on  OutDataTypeStr=Inherit: Same as first input
  SumA31 : Sum  Inputs=|+-  RndMeth=Nearest  SaturateOnIntegerOverflow=on  OutDataTypeStr=Inherit: Same as first input
  SumB21 : Sum  Inputs=|++  RndMeth=Nearest  SaturateOnIntegerOverflow=on  OutDataTypeStr=Inherit: Same as first input
  SumB31 : Sum  Inputs=|++  RndMeth=Nearest  SaturateOnIntegerOverflow=on  OutDataTypeStr=Inherit: Same as first input
  a(2)(1) : Gain  Gain=-1.14298050253990113  ParamDataTypeStr=double  RndMeth=Nearest  SaturateOnIntegerOverflow=on  OutDataTypeStr=Inherit: Same as input
  a(3)(1) : Gain  Gain=0.412801598096188771  ParamDataTypeStr=double  RndMeth=Nearest  SaturateOnIntegerOverflow=on  OutDataTypeStr=Inherit: Same as input
  b(2)(1) : Gain  Gain=2  ParamDataTypeStr=double  RndMeth=Nearest  SaturateOnIntegerOverflow=on  OutDataTypeStr=Inherit: Same as input
  s(1) : Gain  Gain=0.0674552738890718956  ParamDataTypeStr=double  RndMeth=Nearest  SaturateOnIntegerOverflow=on  OutDataTypeStr=Inherit: Same as input
  Output : Outport
  wires:
  Input/1 -> s(1)/1
  s(1)/1 -> SumA21/1
  SumA21/1 -> SumA31/1
  SumA31/1 -> SumB21/1, Delay11/1
  SumB21/1 -> SumB31/1
  SumB31/1 -> Output/1
  a(2)(1)/1 -> SumA21/2
  Delay11/1 -> a(2)(1)/1, b(2)(1)/1, Delay21/1
  b(2)(1)/1 -> SumB21/2
  a(3)(1)/1 -> SumA31/2
  Delay21/1 -> a(3)(1)/1, SumB31/2

== matlab function PPSFB_DC_DC_att_11/MATLAB Function ==
  data: time input; PWM2 output; frequency input; phase input; PWM1 output
function [PWM2,PWM1] = fcn(time,frequency,phase)
Tswitching = 1/frequency; 
PWM1 = 0;
PWM2 = 0; 
y1= mod(time,Tswitching);
if y1<Tswitching/2
    PWM1 = 1; 
end
t_phi = Tswitching*phase/360;
y2 = mod(time+t_phi,Tswitching);
if y2<Tswitching/2
    PWM2 = 1;
end
